simulink model "LAB8ADAsim"  (R2024a)
settings: Solver=VariableStepAuto  StartTime=0.0  StopTime=10.0  RelTol=1e-3
libraries: cstblocks x2, simulink x1
settings Model: Creator=alifuatsakaci  LastModifiedBy=alifuatsakaci
settings RTWCC: GPUComputeCapability=3.5

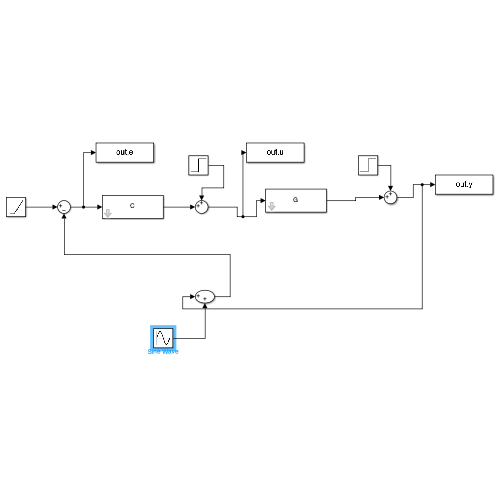
[thumbnail: Simulink's stored preview of the top-level diagram]
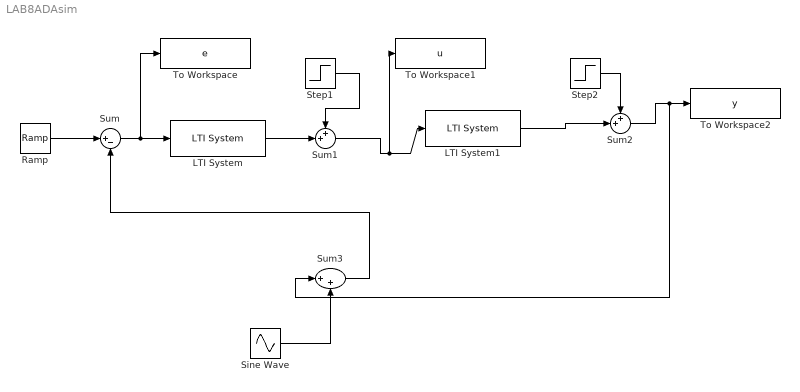
== system LAB8ADAsim ==
  LTI System : cstblocks/LTI System  sys=C  IC=[]  PadeOrder=0
  LTI System1 : cstblocks/LTI System  sys=G  IC=[]  PadeOrder=0
  Ramp : simulink/Sources/Ramp  slope=0  start=0  InitialOutput=0
  Sine Wave : Sin  Amplitude=0.1  Frequency=90  SampleTime=0
  Step1 : Step  Time=0  After=0  SampleTime=0
  Step2 : Step  Time=0  After=0  SampleTime=0
  Sum : Sum  Inputs=|+-
  Sum1 : Sum  Inputs=++|
  Sum2 : Sum  Inputs=++|
  Sum3 : Sum  Inputs=|++
  To Workspace : ToWorkspace  VariableName=e  SaveFormat=Timeseries  SampleTime=-1
  To Workspace1 : ToWorkspace  VariableName=u  SaveFormat=Timeseries  SampleTime=-1
  To Workspace2 : ToWorkspace  VariableName=y  SaveFormat=Timeseries  SampleTime=-1
  wires:
  Ramp/1 -> Sum/1
  Sum/1 -> To Workspace/1, LTI System/1
  Sum1/1 -> To Workspace1/1, LTI System1/1
  Sum2/1 -> To Workspace2/1, Sum3/1
  Sine Wave/1 -> Sum3/2
  LTI System/1 -> Sum1/2
  Step1/1 -> Sum1/1
  LTI System1/1 -> Sum2/2
  Step2/1 -> Sum2/1
  Sum3/1 -> Sum/2
